simulink model "Lab_10_model_1_do_statycznych"  (R2022b)
settings: Solver=VariableStepAuto  StartTime=0.0  StopTime=10.0  RelTol=1e-3
settings Model: Creator=mateu  LastModifiedBy=mateu

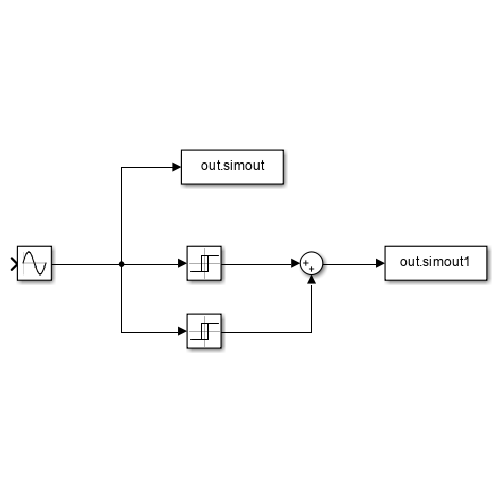
[thumbnail: Simulink's stored preview of the top-level diagram]
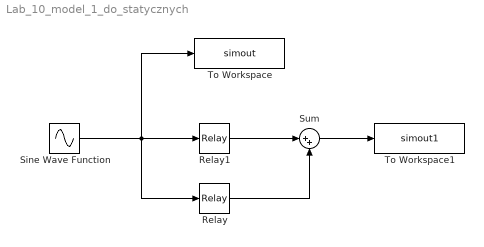
== system Lab_10_model_1_do_statycznych ==
  Relay : Relay
  Relay1 : Relay
  Sine Wave Function : Sin  TimeSource=Use external signal  SampleTime=0
  Sum : Sum  Inputs=|++
  To Workspace : ToWorkspace  VariableName=simout  SaveFormat=Timeseries  SampleTime=-1
  To Workspace1 : ToWorkspace  VariableName=simout1  SaveFormat=Timeseries  SampleTime=-1
  wires:
  Sine Wave Function/1 -> To Workspace/1, Relay/1, Relay1/1
  Relay1/1 -> Sum/1
  Relay/1 -> Sum/2
  Sum/1 -> To Workspace1/1
